simulink model "pid_smithpredictor"  (R2025b)
settings: Solver=VariableStepAuto  StartTime=0.0  StopTime=30  RelTol=1e-3
values from neighbouring files (symbols this model uses):
  kd = gaina(3)    [findkp_ki_kd.m]
  ki = gaina(2)    [findkp_ki_kd.m]
  kp = gaina(1)    [findkp_ki_kd.m]
libraries: cstblocks x2
settings Model: Creator=AIZAZ BADRU  LastModifiedBy=AIZAZ BADRU

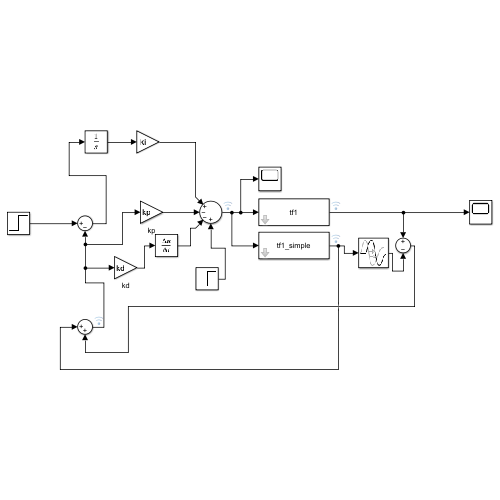
[thumbnail: Simulink's stored preview of the top-level diagram]
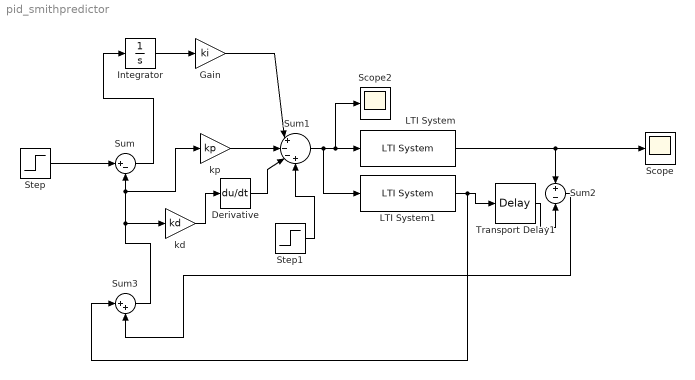
== system pid_smithpredictor ==
  Derivative : Derivative
  Gain : Gain  Gain=ki
  Integrator : Integrator
  LTI System : cstblocks/LTI System  sys=tf1  IC=[]  PadeOrder=0
  LTI System1 : cstblocks/LTI System  sys=tf1_simple  IC=[]  PadeOrder=0
  Scope : Scope
      settings: ActiveDisplayYMinimum=-1  ActiveDisplayYMaximum=1
  Scope2 : Scope
      settings: ActiveDisplayYMinimum=-104.37494526524767  ActiveDisplayYMaximum=36.522581483306922  DataLoggingVariableName=ScopeData2  DataLoggingSaveFormat=Array
  Step : Step  Time=0  After=100  SampleTime=0
  Step1 : Step  Time=7  After=50  SampleTime=0
  Sum : Sum  Inputs=|+-
  Sum1 : Sum  Inputs=|+--+
  Sum2 : Sum  Inputs=+-
  Sum3 : Sum  Inputs=|++
  Transport Delay1 : TransportDelay  DelayTime=0.67
  kd : Gain  Gain=kd
  kp : Gain  Gain=kp
  wires:
  Step/1 -> Sum/1
  kd/1 -> Derivative/1
  kp/1 -> Sum1/2
  Gain/1 -> Sum1/1
  Integrator/1 -> Gain/1
  Sum1/1 -> LTI System1/1, Scope2/1, LTI System/1
  Sum2/1 -> Sum3/2
  Sum3/1 -> kd/1, kp/1, Sum/2
  Sum/1 -> Integrator/1
  Derivative/1 -> Sum1/3
  LTI System/1 -> Sum2/1, Scope/1
  Transport Delay1/1 -> Sum2/2
  LTI System1/1 -> Sum3/1, Transport Delay1/1
  Step1/1 -> Sum1/4
